simulink model "lab1_model2"  (R2012b)
settings: Solver=ode45  StartTime=0.0  StopTime=20.0  RelTol=1e-3
settings Model: Creator=student-at  LastModifiedBy=student-at

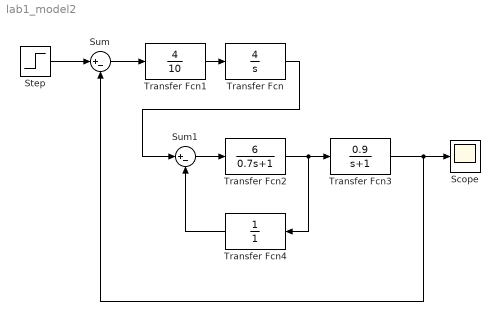
== system lab1_model2 ==
  Scope : Scope
  Step : Step  SampleTime=0
  Sum : Sum  Inputs=|+-
  Sum1 : Sum  Inputs=|+-
  Transfer Fcn : TransferFcn  Numerator=[4]  Denominator=[1 0]
  Transfer Fcn1 : TransferFcn  Numerator=[4]  Denominator=[0 10]
  Transfer Fcn2 : TransferFcn  Numerator=[6]  Denominator=[0.7 1]
  Transfer Fcn3 : TransferFcn  Numerator=[0.9]  Denominator=[1 1]
  Transfer Fcn4 : TransferFcn  Denominator=[0 1]
  wires:
  Step/1 -> Sum/1
  Sum/1 -> Transfer Fcn1/1
  Transfer Fcn1/1 -> Transfer Fcn/1
  Transfer Fcn/1 -> Sum1/1
  Sum1/1 -> Transfer Fcn2/1
  Transfer Fcn2/1 -> Transfer Fcn4/1, Transfer Fcn3/1
  Transfer Fcn3/1 -> Sum/2, Scope/1
  Transfer Fcn4/1 -> Sum1/2
